simulink library "command_converter_lib"  (R2018b)
settings: Solver=VariableStepAuto  StartTime=0.0  StopTime=10.0  RelTol=1e-3
undefined symbols (not defined in the file): DiscIntNeverNeededParam, fswParams, simParams
settings Model: Creator=colem  LastModifiedBy=aact_

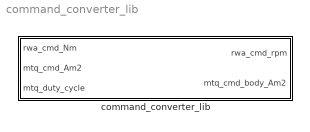
== system command_converter_lib ==
  command_converter_lib : Subsystem  TreatAsAtomicUnit=on
      settings: RTWFcnNameOpts=Use subsystem name  RTWFileNameOpts=Use subsystem name

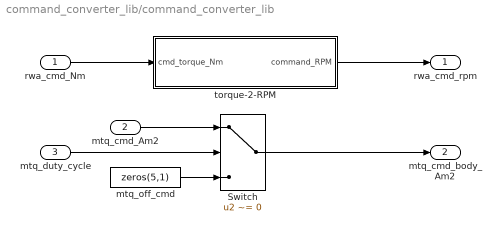
== system command_converter_lib/command_converter_lib ==
  rwa_cmd_Nm : Inport
  mtq_cmd_Am2 : Inport  Port=2
  mtq_duty_cycle : Inport  Port=3
  Switch : Switch  Criteria=u2 ~= 0  OutDataTypeStr=double  InputSameDT=on
  mtq_off_cmd : Constant  Value=zeros(5,1)  OutDataTypeStr=double
  torque-2-RPM : Subsystem
  rwa_cmd_rpm : Outport
  mtq_cmd_body_Am2 : Outport  Port=2
  wires:
  rwa_cmd_Nm/1 -> torque-2-RPM/1(cmd_torque_Nm)
  mtq_cmd_Am2/1 -> Switch/1
  torque-2-RPM/1(command_RPM) -> rwa_cmd_rpm/1
  mtq_duty_cycle/1 -> Switch/2
  mtq_off_cmd/1 -> Switch/3
  Switch/1 -> mtq_cmd_body_Am2/1

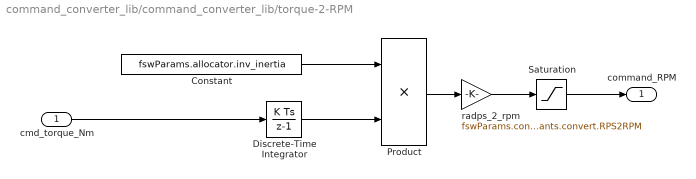
== system command_converter_lib/command_converter_lib/torque-2-RPM ==
  cmd_torque_Nm : Inport
  Constant : Constant  Value=fswParams.allocator.inv_inertia  SampleTime=fswParams.sample_time_s
  Discrete-Time Integrator : DiscreteIntegrator  InitialCondition=simParams.initialConditions.rwa.h_wheel_Nms  SampleTime=-1  ICPrevOutput=DiscIntNeverNeededParam  ICPrevScaledInput=DiscIntNeverNeededParam
  Product : Product
  Saturation : Saturate  UpperLimit=fswParams.allocator.max_RPM  LowerLimit=-fswParams.allocator.max_RPM
  radps_2_rpm : Gain  Gain=fswParams.constants.convert.RPS2RPM
  command_RPM : Outport
  wires:
  Saturation/1 -> command_RPM/1
  Discrete-Time Integrator/1 -> Product/2
  cmd_torque_Nm/1 -> Discrete-Time Integrator/1
  radps_2_rpm/1 -> Saturation/1
  Product/1 -> radps_2_rpm/1
  Constant/1 -> Product/1
